simulink library "mag_mtq_duty_cycle_lib"  (R2018b)
settings: Solver=VariableStepAuto  StartTime=0.0  StopTime=10.0  RelTol=1e-3
undefined symbols (not defined in the file or in its folder): fswParams
libraries: simulink x3
settings Model: Creator=Taylor  LastModifiedBy=Taylor

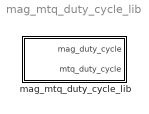
== system mag_mtq_duty_cycle_lib ==
  mag_mtq_duty_cycle_lib : Subsystem

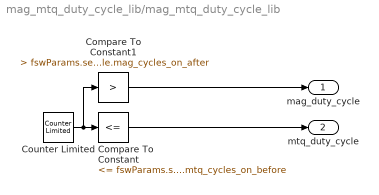
== system mag_mtq_duty_cycle_lib/mag_mtq_duty_cycle_lib ==
  Compare To Constant : simulink/Logic and Bit Operations/Compare To Constant  relop=<=  const=fswParams.sensors.duty_cycle.mtq_cycles_on_before  OutDataTypeStr=boolean
  Compare To Constant1 : simulink/Logic and Bit Operations/Compare To Constant  relop=>  const=fswParams.sensors.duty_cycle.mag_cycles_on_after  OutDataTypeStr=boolean
  Counter Limited : simulink/Sources/Counter Limited  uplimit=fswParams.sensors.duty_cycle.supercycle_length  tsamp=fswParams.sample_time_s
  mag_duty_cycle : Outport
  mtq_duty_cycle : Outport  Port=2
  wires:
  Counter Limited/1 -> Compare To Constant1/1, Compare To Constant/1
  Compare To Constant/1 -> mtq_duty_cycle/1
  Compare To Constant1/1 -> mag_duty_cycle/1
